simulink model "PV_string_model"  (R2019b)
settings: Solver=ode23t  StartTime=0.0  StopTime=8000  RelTol=1e-3
libraries: simulink x1
settings Model: Creator=pimou  LastModifiedBy=pimou

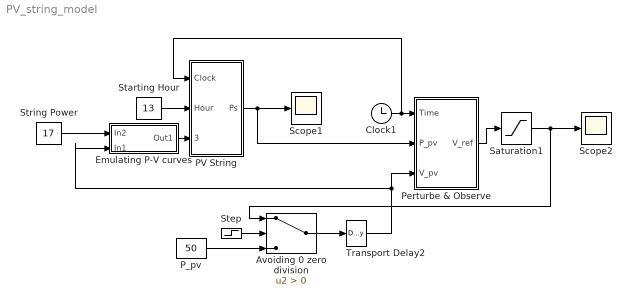
== system PV_string_model ==
  Avoiding 0 zero division : Switch  Criteria=u2 > Threshold
  Clock1 : Clock
  Emulating P-V curves : Subsystem
  PV String : Subsystem  mask{sn=3}
      mask prompts: sn "Season (1=winter, 2=autumn/spring, 3=summer)"
      mask TypeOptions sn: 1 | 2 | 3
  P_pv : Constant  Value=50
  Perturbe & Observe : Subsystem  mask{Tmppt=0.05, Vstep=2}
      mask prompts: Tmppt "T_mppt"; Vstep "V_step"
  Saturation1 : Saturate  UpperLimit=inf  LowerLimit=2
  Scope1 : Scope
  Scope2 : Scope
  Starting Hour : Constant  Value=13
  Step : Step  Time=5  SampleTime=0
  String Power : Constant  Value=17
  Transport Delay2 : TransportDelay  DelayTime=0.001
  wires:
  Starting Hour/1 -> PV String/2(Hour)
  Clock1/1 -> PV String/1(Clock), Perturbe & Observe/1(Time)
  PV String/1(Ps) -> Perturbe & Observe/2(P_pv), Scope1/1
  Perturbe & Observe/1(V_ref) -> Saturation1/1
  Step/1 -> Avoiding 0 zero division/2
  P_pv/1 -> Avoiding 0 zero division/3
  Avoiding 0 zero division/1 -> Transport Delay2/1
  Transport Delay2/1 -> Perturbe & Observe/3(V_pv), Emulating P-V curves/2(In1)
  Saturation1/1 -> Scope2/1, Avoiding 0 zero division/1
  String Power/1 -> Emulating P-V curves/1(In2)
  Emulating P-V curves/1(Out1) -> PV String/3(String P_n)

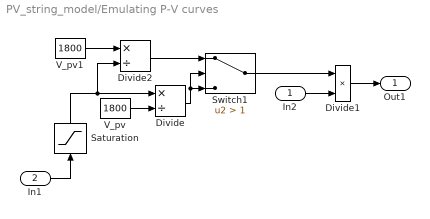
== system PV_string_model/Emulating P-V curves ==
  In2 : Inport
  In1 : Inport  Port=2
  Divide : Product  Inputs=*/
  Divide1 : Product  Inputs=**
  Divide2 : Product  Inputs=*/
  Saturation : Saturate  UpperLimit=inf  LowerLimit=2
  Switch1 : Switch  Criteria=u2 > Threshold  Threshold=1
  V_pv : Constant  Value=1800
  V_pv1 : Constant  Value=1800
  Out1 : Outport
  wires:
  In1/1 -> Saturation/1
  In2/1 -> Divide1/2
  Saturation/1 -> Divide2/2, Divide/1
  Switch1/1 -> Divide1/1
  Divide2/1 -> Switch1/1
  V_pv1/1 -> Divide2/1
  Divide/1 -> Switch1/3, Switch1/2
  V_pv/1 -> Divide/2
  Divide1/1 -> Out1/1

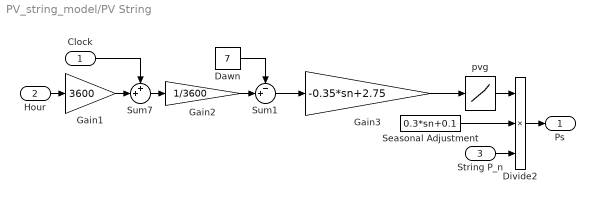
== system PV_string_model/PV String ==
  Clock : Inport
  Hour : Inport  Port=2
  String P_n : Inport  Port=3
  Dawn : Constant  Value=7
  Divide2 : Product  Inputs=3
  Gain1 : Gain  Gain=3600
  Gain2 : Gain  Gain=1/3600
  Gain3 : Gain  Gain=-0.35*sn+2.75
  Seasonal Adjustment : Constant  Value=0.3*sn+0.1
  Sum1 : Sum  Inputs=-+|
  Sum7 : Sum  Inputs=++|
  pvg : Lookup  InputValues="[1   2   3   4   5   6   7   8   9  10  11  12  13  14  15  16  17  18  19  20  21  22  23  24]"  Table="[1.181002      4.7654303      13.969232      31.670729      60.919164      105.05308      167.90074       254.1193      369.76904      523.28521      727.12323      1000.5433      1000.5433      727.12323      523.28521      369.76904       254.1193      167.90074      105.05308      60.919164      31.670729      13.969232      4.7654303       1.181002]"  LookUpMeth=Interpolation-Use End Values
  Ps : Outport
  wires:
  Seasonal Adjustment/1 -> Divide2/2
  String P_n/1 -> Divide2/3
  Divide2/1 -> Ps/1
  Hour/1 -> Gain1/1
  Clock/1 -> Sum7/1
  Gain1/1 -> Sum7/2
  Sum7/1 -> Gain2/1
  Sum1/1 -> Gain3/1
  Gain2/1 -> Sum1/2
  Dawn/1 -> Sum1/1
  Gain3/1 -> pvg/1
  pvg/1 -> Divide2/1

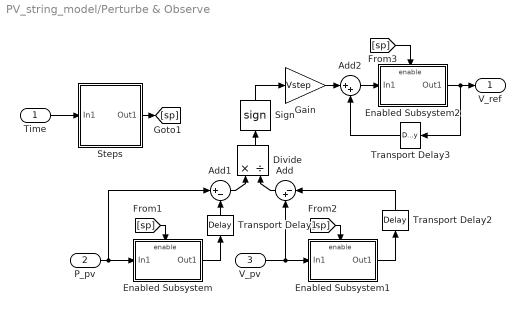
== system PV_string_model/Perturbe & Observe ==
  Time : Inport
  P_pv : Inport  Port=2
  V_pv : Inport  Port=3
  Add : Sum  Inputs=|-+
  Add1 : Sum  Inputs=|+-
  Add2 : Sum  Inputs=|++
  Divide : Product  Inputs=*/
  Enabled Subsystem : Subsystem  TreatAsAtomicUnit=on
  Enabled Subsystem1 : Subsystem  TreatAsAtomicUnit=on
  Enabled Subsystem2 : Subsystem  TreatAsAtomicUnit=on
  Gain : Gain  Gain=Vstep
  Sign : Signum
  Steps : Subsystem
  Transport Delay1 : TransportDelay  DelayTime=0.001
  Transport Delay2 : TransportDelay  DelayTime=0.001
  Transport Delay3 : TransportDelay  DelayTime=0.001
  V_ref : Outport
  wires:
  Enabled Subsystem/1(Out1) -> Transport Delay1/1
  Divide/1 -> Sign/1
  Add/1 -> Divide/2
  V_pv/1 -> Add/2, Enabled Subsystem1/1(In1)
  Add1/1 -> Divide/1
  Enabled Subsystem1/1(Out1) -> Transport Delay2/1
  Transport Delay1/1 -> Add1/2
  [sp] -> Enabled Subsystem1/Enable
  Time/1 -> Steps/1(In1)
  Steps/1(Out1) -> [sp]
  [sp] -> Enabled Subsystem2/Enable
  Gain/1 -> Add2/1
  P_pv/1 -> Add1/1, Enabled Subsystem/1(In1)
  Sign/1 -> Gain/1
  [sp] -> Enabled Subsystem/Enable
  Transport Delay2/1 -> Add/1
  Enabled Subsystem2/1(Out1) -> Transport Delay3/1, V_ref/1
  Add2/1 -> Enabled Subsystem2/1(In1)
  Transport Delay3/1 -> Add2/2

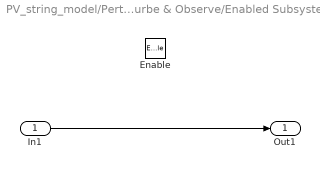
== system PV_string_model/Perturbe & Observe/Enabled Subsystem ==
  In1 : Inport
  Enable : EnablePort
  Out1 : Outport
  wires:
  In1/1 -> Out1/1

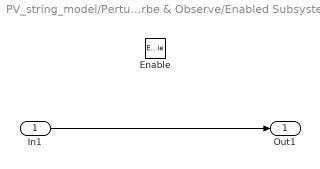
== system PV_string_model/Perturbe & Observe/Enabled Subsystem1 ==
  In1 : Inport
  Enable : EnablePort
  Out1 : Outport
  wires:
  In1/1 -> Out1/1

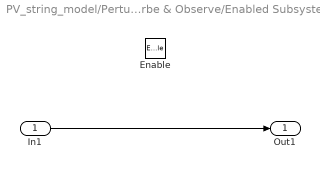
== system PV_string_model/Perturbe & Observe/Enabled Subsystem2 ==
  In1 : Inport
  Enable : EnablePort
  Out1 : Outport
  wires:
  In1/1 -> Out1/1

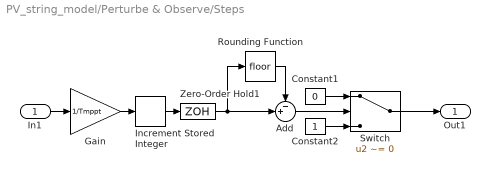
== system PV_string_model/Perturbe & Observe/Steps ==
  In1 : Inport
  Add : Sum  Inputs=-+|
  Constant1 : Constant  Value=0
  Constant2 : Constant
  Gain : Gain  Gain=1/Tmppt
  Increment Stored Integer : simulink/Additional Math & Discrete/Additional Math: Increment - Decrement/Increment Stored Integer
      settings: SourceProductName=Simulink
  Rounding Function : Rounding
  Switch : Switch  Criteria=u2 ~= 0
  Zero-Order Hold1 : ZeroOrderHold  SampleTime=1/10000
  Out1 : Outport
  wires:
  In1/1 -> Gain/1
  Add/1 -> Switch/2
  Switch/1 -> Out1/1
  Constant1/1 -> Switch/1
  Gain/1 -> Increment Stored Integer/1
  Rounding Function/1 -> Add/1
  Zero-Order Hold1/1 -> Add/2, Rounding Function/1
  Constant2/1 -> Switch/3
  Increment Stored Integer/1 -> Zero-Order Hold1/1
